simulink model "blockdemo"  (Simulink 6.3)
settings: Solver=FixedStepDiscrete  StartTime=0.0  StopTime=16.0  RelTol=1e-3
InitFcn:
  | %% DSPBuilder Start
  | alt_dspbuilder_update_model(bdroot)
  | %% DSPBuilder End
libraries: allblocks_alteradspbuilder2 x12
settings Model: LastModifiedBy=delphick

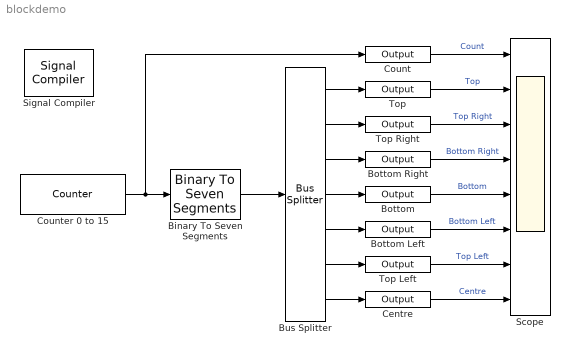
== system blockdemo ==
  Binary To Seven Segments : allblocks_alteradspbuilder2/Binary To Seven Segments
  Bottom : allblocks_alteradspbuilder2/Output  iofile=C:\workspace_clean\Documentation\DesignExamples\Tutorials\UnitBlocks\GateAndControl\BinaryToSevenSegments\tb_blockdemo\blockdemo_Bottom.capture  BusType=Single Bit  bwl=8  bwr=0  PORTTYPE=Output
  Bottom Left : allblocks_alteradspbuilder2/Output  iofile=C:\workspace_clean\Documentation\DesignExamples\Tutorials\UnitBlocks\GateAndControl\BinaryToSevenSegments\tb_blockdemo\blockdemo_Bottom+Left.capture  BusType=Single Bit  bwl=8  bwr=0  PORTTYPE=Output
  Bottom Right : allblocks_alteradspbuilder2/Output  iofile=C:\workspace_clean\Documentation\DesignExamples\Tutorials\UnitBlocks\GateAndControl\BinaryToSevenSegments\tb_blockdemo\blockdemo_Bottom+Right.capture  BusType=Single Bit  bwl=8  bwr=0  PORTTYPE=Output
  Bus Splitter : allblocks_alteradspbuilder2/Bus Splitter  BusType=Unsigned Integer  bwl=7  bwr=0
  Centre : allblocks_alteradspbuilder2/Output  iofile=C:\workspace_clean\Documentation\DesignExamples\Tutorials\UnitBlocks\GateAndControl\BinaryToSevenSegments\tb_blockdemo\blockdemo_Centre.capture  BusType=Single Bit  bwl=8  bwr=0  PORTTYPE=Output
  Count : allblocks_alteradspbuilder2/Output  iofile=C:\workspace_clean\Documentation\DesignExamples\Tutorials\UnitBlocks\GateAndControl\BinaryToSevenSegments\tb_blockdemo\blockdemo_Count.capture  BusType=Unsigned Integer  bwl=4  bwr=0  PORTTYPE=Output
  Counter 0 to 15 : allblocks_alteradspbuilder2/Counter  BusType=Unsigned Integer  bwl=4  bwr=0  use_modulo=on  modulo=16  SpecifyClock=off  direction=Increment  use_sload=off  use_sset=off  svalue=1  use_ena=off  use_sclr=off
  Scope : Scope  NumInputPorts=8
      settings: TimeRange=16  YMin=0~-2~-2~-2~-2~-2~-2~-2  YMax=16~2~2~2~2~2~2~2
  Signal Compiler : allblocks_alteradspbuilder2/Signal Compiler  DeviceFamily=Stratix IV  DeviceName=AUTO  EnableSignalTap=off  SignalTapDepth=128  UseBoardBlock=off  StpUseDefaultClock=on  StpClock=clock
  Top : allblocks_alteradspbuilder2/Output  iofile=C:\workspace_clean\Documentation\DesignExamples\Tutorials\UnitBlocks\GateAndControl\BinaryToSevenSegments\tb_blockdemo\blockdemo_Top.capture  BusType=Single Bit  bwl=8  bwr=0  PORTTYPE=Output
  Top Left : allblocks_alteradspbuilder2/Output  iofile=C:\workspace_clean\Documentation\DesignExamples\Tutorials\UnitBlocks\GateAndControl\BinaryToSevenSegments\tb_blockdemo\blockdemo_Top+Left.capture  BusType=Single Bit  bwl=8  bwr=0  PORTTYPE=Output
  Top Right : allblocks_alteradspbuilder2/Output  iofile=C:\workspace_clean\Documentation\DesignExamples\Tutorials\UnitBlocks\GateAndControl\BinaryToSevenSegments\tb_blockdemo\blockdemo_Top+Right.capture  BusType=Single Bit  bwl=8  bwr=0  PORTTYPE=Output
  wires:
  Counter 0 to 15/1 -> Binary To Seven Segments/1, Count/1
  Binary To Seven Segments/1 -> Bus Splitter/1
  Bus Splitter/1 -> Top/1
  Bus Splitter/7 -> Centre/1
  Bus Splitter/4 -> Bottom/1
  Bus Splitter/2 -> Top Right/1
  Bus Splitter/3 -> Bottom Right/1
  Bus Splitter/5 -> Bottom Left/1
  Bus Splitter/6 -> Top Left/1
  Count/1 -> Scope/1  "Count"
  Top/1 -> Scope/2  "Top"
  Top Right/1 -> Scope/3  "Top Right"
  Bottom Right/1 -> Scope/4  "Bottom Right"
  Bottom/1 -> Scope/5  "Bottom"
  Bottom Left/1 -> Scope/6  "Bottom Left"
  Top Left/1 -> Scope/7  "Top Left"
  Centre/1 -> Scope/8  "Centre"
